simulink model "symulacja"  (R2021b)
settings: Solver=FixedStepDiscrete  StartTime=0.0  StopTime=30  FixedStep=0.08  RelTol=1e-3
values from neighbouring files (symbols this model uses):
  R = [1 -0.446274503438 -0.477535408753 -0.0761900878093]    [inne_RST.mat]    (also in pomiary.mat = [1 -0.580488001034 -0.378788059627 -0.040723939339]; pzpd.m = R/R(1); variables_pzpd.mat = [1 -0.55004580731 -0.401109305745 -0.0488448869454])
  S = [-80.0099887925 221.853468864 -205.194634947 63.2491401531]    [inne_RST.mat]    (also in pomiary.mat = [110239.549362 -325281.560403 319945.729545 -104903.058534]; pzpd.m = S/R(1); variables_pzpd.mat = [1457608.23927 -4241257.79416 4114804.22785 -1331082.00051])
  T = [-0.68009814706 0.578083425001]    [inne_RST.mat]    (also in pomiary.mat = [4.39979800589 -3.73982830501]; pzpd.m = T/R(1); variables_pzpd.mat = [726.724582158 -654.052123942])
undefined symbols (not defined in the file or in its folder): Amc, Bmc, sigbuilder_block
settings Model: Creator=STUDENT  LastModifiedBy=STUDENT

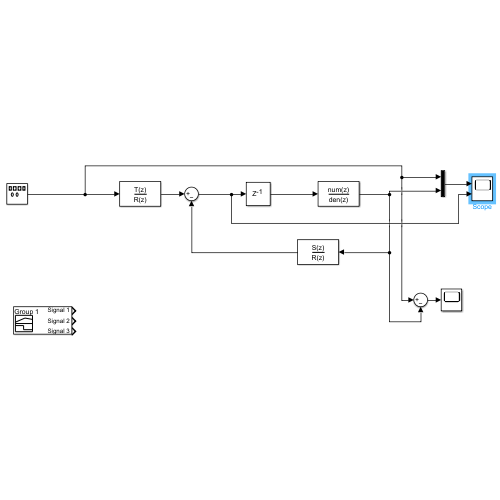
[thumbnail: Simulink's stored preview of the top-level diagram]
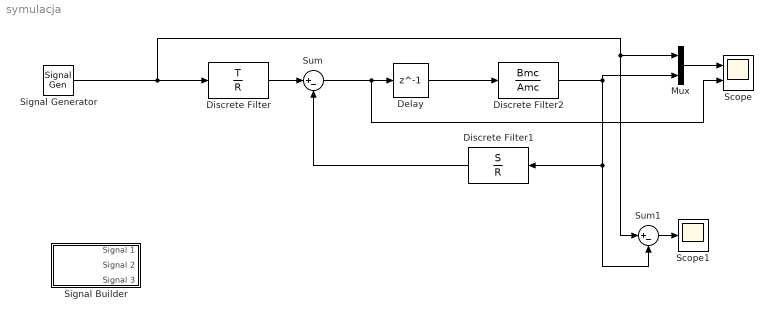
== system symulacja ==
  Delay : Delay  DelayLength=1
  Discrete Filter : DiscreteFilter  Numerator=T  Denominator=R
  Discrete Filter1 : DiscreteFilter  Numerator=S  Denominator=R
  Discrete Filter2 : DiscreteFilter  Numerator=Bmc  Denominator=Amc
  Mux : Mux  Inputs=2
  Scope : Scope  NumInputPorts=2
  Scope1 : Scope
  Signal Generator : SignalGenerator  WaveForm=square  Amplitude=5 * pi /180  Frequency=1/10
  Signal Builder : Subsystem  Tag=STV Subsys  LoadFcn=sigbuilder_block('load');  StartFcn=sigbuilder_block('start');  StopFcn=sigbuilder_block('stop');  ClipboardFcn=sigbuilder_block('clipboard');  mask(Sigbuilder block){tuvar=[0:10]}
      mask help: Simulink:masks:SigbuilderBlock_MD
      mask init:
      | if ~strcmp(get_param(bdroot(gcbh),'SimulationStatus'),'stopped') tuvar = sigbuilder_block('maskInit'); end
      settings: CopyFcn=sigbuilder_block('copy');  DeleteFcn=sigbuilder_block('delete');  ModelCloseFcn=sigbuilder_block('modelClose');  PreSaveFcn=sigbuilder_block('preSave');  PauseFcn=sigbuilder_block('pause');  ContinueFcn=sigbuilder_block('continue');  NameChangeFcn=sigbuilder_block('namechange');  OpenFcn=sigbuilder_block('open',[314.25 165 550.5 399.75 ]);  CloseFcn=sigbuilder_block('close');
      mask Display: plot(0, 0, 100, 100,[2, 2, 32, 32, 2], [68, 8, 8, 68, 68],[32, 2], [38, 38], [32, 19, 2],[53, 60, 44], [32, 17, 17, 2],[16, 16, 31, 31]);txt = getActiveGroup(gcbh);text(2, 100, txt,'verticalAlignment', 'top');
  Sum : Sum  Inputs=|+-
  Sum1 : Sum  Inputs=|+-
  wires:
  Discrete Filter/1 -> Sum/1
  Discrete Filter1/1 -> Sum/2
  Discrete Filter2/1 -> Sum1/2, Discrete Filter1/1, Mux/2
  Sum/1 -> Scope/2, Delay/1
  Delay/1 -> Discrete Filter2/1
  Signal Generator/1 -> Sum1/1, Mux/1, Discrete Filter/1
  Sum1/1 -> Scope1/1
  Mux/1 -> Scope/1

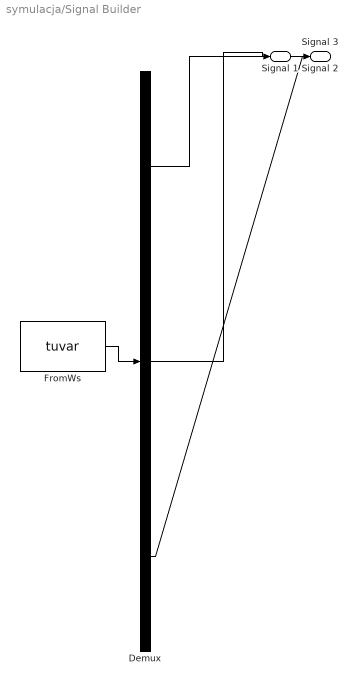
== system symulacja/Signal Builder ==
  Demux : Demux  Tag=STV Demux  Outputs=3
      settings: DisplayOption=none
  FromWs : FromWorkspace  Tag=STV FromWs  VariableName=tuvar
      SigBuilderData=|
      | common.afterFinalStr = 'Extrapolate'
      | common.sampleTime = 0
      | dataSet.timeRange = [0 80]
      | dataSet.name = 'Group 1'
      | sbobj.Groups.Name = 'Group 1'
      | sbobj.Groups.Signals(1).Name = 'Signal 1'
      | sbobj.Groups.Signals(1).XData = [0 5 5 10 10 15 15 20 20 25 25 30 30 35 35 40 40 45 45 50 50 55 55 60 60 65 65 70 70 75 75 80]
      | sbobj.Groups.Signals(1).YData = [0.1 0.1 -0.1 -0.1 0.2 0.2 -0.2 -0.2 0.3 0.3 -0.3 -0.3 0.4 0.4 -0.4 -0.4 0.5 0.5 -0.5 -0.5 0.6 0.6 -0.6 -0.6 0.7 0.7 -0.7 -0.7 0.8 0.8 -0.8 -0.8]
      | sbobj.Groups.Signals(2).Name = 'Signal 2'
      | sbobj.Groups.Signals(2).XData = [0 5 5 10 10 15 15 20 20 25 25 30 30 35 35 40 40 45 45 50 50 55 55 60 60 65 65 70 70 75 75 80]
      | sbobj.Groups.Signals(2).YData = [0 0.1 0 -0.1 0 0.2 0 -0.2 0 0.3 0 -0.3 0 0.4 0 -0.4 0 0.5 0 -0.5 0 0.6 0 -0.6 0 0.7 0 -0.7 0 0.8 0 -0.8]
      | sbobj.Groups.Signals(3).Name = 'Signal 3'
      | sbobj.Groups.Signals(3).XData = [0 10 10 20 20 30 30 40 40 50 50 60 60 70 70 80]
      | sbobj.Groups.Signals(3).YData = [0.1 0.1 -0.1 -0.1 0.2 0.2 -0.2 -0.2 0.3 0.3 -0.3 -0.3 0.4 0.4 -0.4 -0.4]
      | sbobj.Groups.TimeRange = [0 80]
  Signal 1 : Outport  Tag=STV Outport
  Signal 2 : Outport  Tag=STV Outport  Port=2
  Signal 3 : Outport  Tag=STV Outport  Port=3
  wires:
  FromWs/1 -> Demux/1
  Demux/1 -> Signal 1/1
  Demux/2 -> Signal 2/1
  Demux/3 -> Signal 3/1
